simulink model "boucing_ball1"  (R2022a)
settings: Solver=VariableStepAuto  StartTime=0.0  StopTime=10.0  RelTol=1e-3
libraries: vrlib x2
settings Model: Creator=Vivianne  LastModifiedBy=Vivianne
settings ModelReferenceCC: EnableRefExpFcnMdlSchedulingChecks=off
settings RTWCC: Description=Generic Real-Time Target

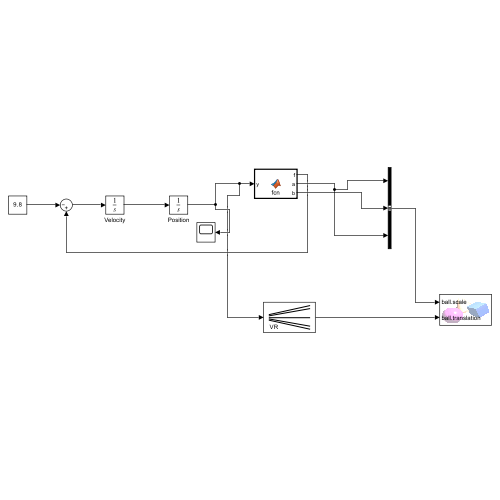
[thumbnail: Simulink's stored preview of the top-level diagram]
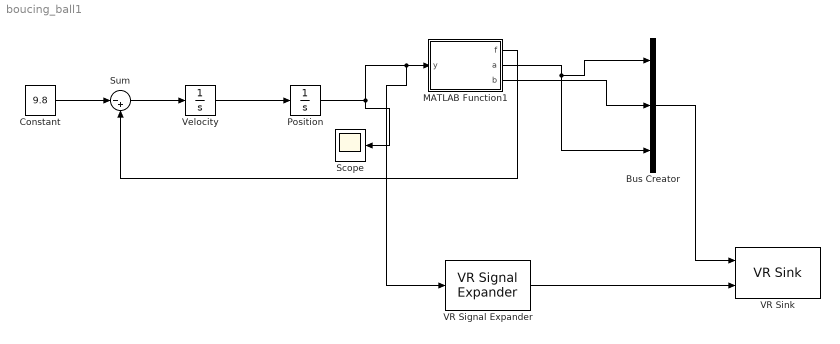
== system boucing_ball1 ==
  Bus Creator : BusCreator  Inputs=3
  Constant : Constant  Value=9.8
  MATLAB Function1 : MATLAB Function  TreatAsAtomicUnit=on
  Position : Integrator  InitialCondition=20
  Scope : Scope
  Sum : Sum  Inputs=|-+
  VR Signal Expander : vrlib/VR Signal Expander  outwidth=3  outidx=[2]
  VR Sink : vrlib/VR Sink  InstantiateOnLoad=on  SampleTime=0.01  ViewEnable=on  RemoteChange=off  RemoteView=off  FieldsWritten=ball.scale.3.1.1.double#ball.translation.3.1.1.double  WorldFileName=boucing-ball2.x3d  AutoView=off  VideoDimensions=[]  AllowVariableSize=off
  Velocity : Integrator
  wires:
  Velocity/1 -> Position/1
  Position/1 -> VR Signal Expander/1, MATLAB Function1/1(y), Scope/1
  Constant/1 -> Sum/1
  Sum/1 -> Velocity/1
  MATLAB Function1/1(f) -> Sum/2
  VR Signal Expander/1 -> VR Sink/2
  MATLAB Function1/2(a) -> Bus Creator/3, Bus Creator/1
  Bus Creator/1 -> VR Sink/1
  MATLAB Function1/3(b) -> Bus Creator/2

== matlab function boucing_ball1/MATLAB Function1 ==
  data: y input; f output; a output; b output
function [f, a, b] = fcn(y)
%#eml

if y<1e-4;
    y=1e-4
end

if y<1.5
    f=500*(1.5-y)
    a=sqrt(1.5^3/y);
    b=y;
else 
    f=0;
    a=1.5;
    b=1.5
end
